simulink model "WPS_system_n_mppt"  (R2019b)
settings: Solver=VariableStepAuto  StartTime=0.0  StopTime=10.0  RelTol=1e-3
undefined symbols (not defined in the file or in its folder): Acid, Lead
libraries: powerlib x17, electricdrivelib x1, powerlib_meascontrol x1, re_lib x1
settings Model: Creator=root  LastModifiedBy=root

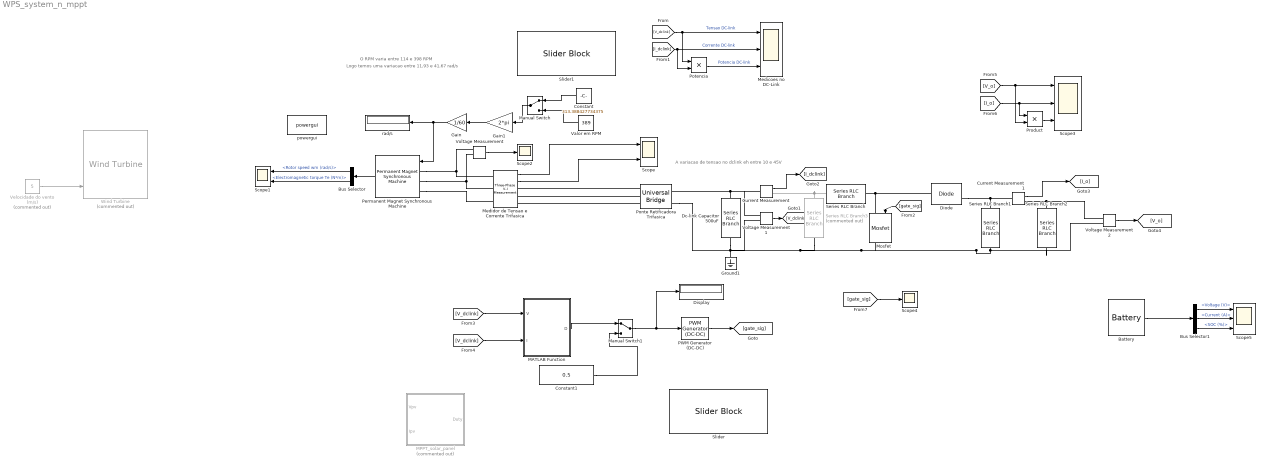
== system WPS_system_n_mppt ==
  note: A variacao de tensao no dclink eh entre 10 e 45V
  note: Logo temos uma variacao entre 11,93 e 41,67 rad/s
  note: O RPM varia entre 114 e 398 RPM
  Battery : electricdrivelib/Extra Sources/Battery  BatType=Lead-Acid  ShowTempParam=off  ThermalPreset=no  ShowAgeParam=off  NomV=12  NomQ=100  SOC=10  Batt_Tr=30  PresetModel=on  MaxQ=104.1667  MinV=9  FullV=13.0658  Dis_rate=20  R=0.0012  Normal_OP=31.0278  expZone="[12.2171     0.333333]"  current=[6.5 13 32.5]  Units=Time  Tci=20  NomT=20  T2=-30  MaxQ2=4.8  FullV2=7.1  Normal_OP2=5.655  expZone2="[6.58           1]"  Rca=0.6  ti=2000  Dp=0  Neq0=0  Tsim=1e6  Ta1=25  Qeol=5.4*0.9  Reol=0.013333*1.2  Char_age=[2.3478, 3]  Dis_age=[2.3478, 10]  N1=1500  N2=10500  N3=1000  N4=1400  Ta2=45  N5=950
      settings: SourceProductName=Simscape Electrical
  Bus Selector : BusSelector  OutputSignals=Rotor speed wm (rad/s),Electromagnetic torque Te (N*m)
  Bus Selector1 : BusSelector  OutputSignals=Voltage (V),Current (A),SOC (%)
  Constant : Constant  Value=313.388427734375
  Constant1 : Constant  Value=0.5
  Current Measurement : powerlib/Measurements/Current Measurement  PhasorSimulation=off  OutputType=Complex  PSBequivalent=0
      settings: SourceProductName=Simscape Electrical
  Current Measurement1 : powerlib/Measurements/Current Measurement  PhasorSimulation=off  OutputType=Complex  PSBequivalent=0
      settings: SourceProductName=Simscape Electrical
  Dc-link Capacitor 500uF : powerlib/Elements/Series RLC Branch  LConnTagsString=__new0  RConnTagsString=__new0  BranchType=C  Resistance=1  Inductance=1e-3  SetiL0=off  InitialCurrent=0  Capacitance=1000e-6  Setx0=off  InitialVoltage=0  Measurements=None
      settings: SourceProductName=Simscape Electrical
  Diode : powerlib/Power Electronics/Diode  Ron=0.001  Lon=0  Vf=0.7  IC=0  UseSnubber=0  Rs=500  Cs=250e-9  Measurements=on
      settings: SourceProductName=Simscape Electrical
  Display : Display
  Gain : Gain  Gain=1/60
  Gain1 : Gain  Gain=2*pi
  Ground1 : powerlib/Elements/Ground  LConnTagsString=a
      settings: SourceProductName=Simscape Electrical
  MATLAB Function : MATLAB Function  TreatAsAtomicUnit=on
  "MPPT_solar_panel " : MATLAB Function  Commented=on  TreatAsAtomicUnit=on
  Manual Switch : ManualSwitch
  Manual Switch1 : ManualSwitch
  Medicoes no DC-Link : Scope  NumInputPorts=3
  Medidor de Tensao e Corrente Trifasica : powerlib/Measurements/Three-Phase V-I Measurement  VoltageMeasurement=phase-to-ground  SetLabelV=off  LabelV=Vabc  Vpu=off  VpuLL=off  CurrentMeasurement=yes  SetLabelI=off  LabelI=Iabc  Ipu=off  Pbase=100e6  Vbase=500e3  OutputType=Complex  PhasorSimulation=off  PSBequivalent=0
      settings: SourceProductName=Simscape Electrical
  Mosfet : powerlib/Power Electronics/Mosfet  Ron=0.1  Lon=0  Rd=0.01  Vfd=0  IC=0  Rs=1e5  Cs=inf  Measurements=on
      settings: SourceProductName=Simscape Electrical
  PWM Generator (DC-DC) : powerlib_meascontrol/Pulse & Signal Generators/PWM Generator (DC-DC)  Fsw=50e3  Ts=0
      settings: SourceProductName=Simscape Electrical
  "Permanent Magnet Synchronous Machine " : powerlib/Machines/Permanent Magnet Synchronous Machine  NbPhases=3  FluxDistribution=Sinusoidal  RotorType=Round  MechanicalLoad=Speed w  PresetModel=No  ShowDetailedParameters=on  MeasurementBus=off  Resistance=0.18  Inductance=8.5e-3  dqInductances=[8.5e-3,8.5e-3]  La=0.000835  MachineConstant=Flux linkage established by magnets (V.s)  Flux=0.186667  VoltageCst=101.5729  TorqueCst=0.84  Flat=120  Mechanical=[0.00038 0.000303448 8]  PolePairs=3  InitialConditions=[0,0, 0,0]  InitialConditions5ph=[0 0 0 0 0 0]  RefAngle=90 degrees behind phase A axis (modified Park)  IterativeDiscreteModel=Trapezoidal non iterative  TsBlock=-1  TsPowergui=0
  Ponte Retificadora Trifasica : powerlib/Power Electronics/Universal Bridge  Arms=3  SnubberResistance=1e4  SnubberCapacitance=100e-6  Device=Diodes  Ron=1e-5  Lon=0  ForwardVoltages="[  0  0  ]"  ForwardVoltage=0  GTOparameters=[ 10e-6 , 20e-6 ]  IGBTparameters=[ 1e-6 , 2e-6 ]  Measurements=None  Measurements_2=None  converterType=Rectifier
      settings: SourceProductName=Simscape Electrical
  Potencia : Product
  Product : Product
  Scope : Scope  NumInputPorts=2
  Scope1 : Scope  NumInputPorts=2
  Scope2 : Scope
  Scope3 : Scope  NumInputPorts=3
  Scope4 : Scope
  Scope5 : Scope  NumInputPorts=3
  Series RLC Branch : powerlib/Elements/Series RLC Branch  LConnTagsString=__new0  RConnTagsString=__new0  BranchType=L  Resistance=1  Inductance=2.7e-3  SetiL0=off  InitialCurrent=0  Capacitance=1e-6  Setx0=off  InitialVoltage=0  Measurements=None
      settings: SourceProductName=Simscape Electrical
  Series RLC Branch1 : powerlib/Elements/Series RLC Branch  LConnTagsString=__new0  RConnTagsString=__new0  BranchType=RC  Resistance=1e-4  Inductance=1e-3  SetiL0=off  InitialCurrent=0  Capacitance=1000e-6  Setx0=off  InitialVoltage=0  Measurements=None
      settings: SourceProductName=Simscape Electrical
  Series RLC Branch2 : powerlib/Elements/Series RLC Branch  LConnTagsString=__new0  RConnTagsString=__new0  BranchType=R  Resistance=10  Inductance=1e-3  SetiL0=off  InitialCurrent=0  Capacitance=1000e-6  Setx0=off  InitialVoltage=0  Measurements=None
      settings: SourceProductName=Simscape Electrical
  Series RLC Branch3 : powerlib/Elements/Series RLC Branch  Commented=on  LConnTagsString=__new0  RConnTagsString=__new0  BranchType=R  Resistance=10  Inductance=1e-3  SetiL0=off  InitialCurrent=0  Capacitance=1000e-6  Setx0=off  InitialVoltage=0  Measurements=None
      settings: SourceProductName=Simscape Electrical
  Slider : SliderBlock  ScaleMax=1
  Slider1 : SliderBlock  ScaleMin=114  ScaleMax=389
  Valor em RPM : Constant  Value=389
  Velocidade do vento (m/s) : Constant  Commented=on  Value=5
  Voltage Measurement : powerlib/Measurements/Voltage Measurement  PhasorSimulation=off  OutputType=Complex  PSBequivalent=0
      settings: SourceProductName=Simscape Electrical
  Voltage Measurement1 : powerlib/Measurements/Voltage Measurement  PhasorSimulation=off  OutputType=Complex  PSBequivalent=0
      settings: SourceProductName=Simscape Electrical
  Voltage Measurement2 : powerlib/Measurements/Voltage Measurement  PhasorSimulation=off  OutputType=Complex  PSBequivalent=0
      settings: SourceProductName=Simscape Electrical
  Wind Turbine : re_lib/Wind Generation/Wind Turbine  Commented=on  Pnom=1.1e3  Pelec_base=1.1e3/0.9  wind_base=5  P_wind_base=0.8  speed_nom=1  pitch_angle=0  c1_c6="[0.51763          116          0.4            5           21     0.006795]"  cp_nom=0.48  lambda_nom=8.1
      settings: SourceProductName=Simscape Electrical  SourceProductBaseCode=PS
  powergui : powerlib/powergui  Priority=1  SimulationMode=Discrete  SampleTime=10e-6  frequency=60  Iterations=50  frequencyindice=0  Pbase=100e6  ErrMax=1e-4  UnitsV=kV  UnitsW=MW  buscounter=0  FunctionMessages=off  echomessages=off  EnableUseOfTLC=off  CurrentSourceSwitches=off  DisableSnubberDevices=off  DisableRonSwitches=off  DisableVfSwitches=off  DisplayEquations=off  AutomaticDiscreteSolvers=off  SolverType=Tustin/Backward Euler (TBE)  Interpol=off  ExternalGateDelay=off  methode=off  Ts=100  x0status=blocks  SPID=on  SwTol=0  HookPort=off  NonlinearTolerance=1e-4  nMaxIteration=100  ContinueOnMaxIteration=off  RestoreLinks=warning  ResistiveCurrentMeasurement=off  Frange=[0:2:500]  Ylog=off  Xlog=on  ShowGrid=off  save=off  variable=ZData  structure=0  ZoomFFT=off  StartTime=0.0  cycles=1  DisplayStyle=1  fundamental=60  FreqAxis=off  MaxFrequency=1000  frequencyindicesteady=1  RmsSteady=1  display=off
      settings: SourceProductName=Simscape Electrical
  rad/s : Display
  wires:
  Velocidade do vento (m/s)/1 -> Wind Turbine/3
  Medidor de Tensao e Corrente Trifasica/1 -> Scope/1
  Medidor de Tensao e Corrente Trifasica/2 -> Scope/2
  "Permanent Magnet Synchronous Machine "/1 -> Bus Selector/1
  Voltage Measurement/1 -> Scope2/1
  PWM Generator (DC-DC)/1 -> [gate_sig]
  Bus Selector/1 -> Scope1/1  "<Rotor speed wm (rad/s)>"
  Bus Selector/2 -> Scope1/2  "<Electromagnetic torque Te (N*m)>"
  Gain1/1 -> Gain/1
  Gain/1 -> rad/s/1, "Permanent Magnet Synchronous Machine "/1
  Valor em RPM/1 -> Manual Switch/2
  Manual Switch/1 -> Gain1/1
  Voltage Measurement1/1 -> [V_dclink]
  Current Measurement/1 -> [I_dclink]
  [V_dclink] -> Medicoes no DC-Link/1, Potencia/1  "Tensao DC-link"
  [I_dclink] -> Medicoes no DC-Link/2, Potencia/2  "Corrente DC-link"
  Potencia/1 -> Medicoes no DC-Link/3  "Potencia DC-link"
  [gate_sig] -> Mosfet/1
  Current Measurement1/1 -> [I_o]
  Voltage Measurement2/1 -> [V_o]
  [V_o] -> Product/2, Scope3/1
  [I_o] -> Product/1, Scope3/2
  Product/1 -> Scope3/3
  [gate_sig] -> Scope4/1
  [V_dclink] -> MATLAB Function/1(V)
  [V_dclink] -> MATLAB Function/2(I)
  Manual Switch1/1 -> Display/1, PWM Generator (DC-DC)/1
  MATLAB Function/1(D) -> Manual Switch1/1
  Constant1/1 -> Manual Switch1/2
  Constant/1 -> Manual Switch/1
  Battery/1 -> Bus Selector1/1
  Bus Selector1/2 -> Scope5/2  "<Current (A)>"
  Bus Selector1/1 -> Scope5/1  "<Voltage (V)>"
  Bus Selector1/3 -> Scope5/3  "<SOC (%)>"
  connections:
  "Permanent Magnet Synchronous Machine "/LConn1 -- Voltage Measurement/LConn1 -- Medidor de Tensao e Corrente Trifasica/LConn1
  "Permanent Magnet Synchronous Machine "/LConn2 -- Medidor de Tensao e Corrente Trifasica/LConn2 -- Voltage Measurement/LConn2
  "Permanent Magnet Synchronous Machine "/LConn3 -- Medidor de Tensao e Corrente Trifasica/LConn3
  Ponte Retificadora Trifasica/LConn1 -- Medidor de Tensao e Corrente Trifasica/RConn1
  Ponte Retificadora Trifasica/LConn2 -- Medidor de Tensao e Corrente Trifasica/RConn2
  Ponte Retificadora Trifasica/LConn3 -- Medidor de Tensao e Corrente Trifasica/RConn3
  Ground1/LConn1 -- Ponte Retificadora Trifasica/RConn2 -- Voltage Measurement1/LConn2 -- Voltage Measurement2/LConn2 -- Series RLC Branch2/RConn1 -- Series RLC Branch1/RConn1 -- Mosfet/RConn1 -- Series RLC Branch3/RConn1 -- Dc-link Capacitor 500uF/RConn1
  Dc-link Capacitor 500uF/LConn1 -- Current Measurement/LConn1 -- Voltage Measurement1/LConn1 -- Ponte Retificadora Trifasica/RConn1
  Mosfet/LConn1 -- Diode/LConn1 -- Series RLC Branch/RConn1
  Diode/RConn1 -- Current Measurement1/LConn1 -- Series RLC Branch1/LConn1
  Current Measurement1/RConn1 -- Series RLC Branch2/LConn1 -- Voltage Measurement2/LConn1
  Series RLC Branch3/LConn1 -- Series RLC Branch/LConn1 -- Current Measurement/RConn1

== matlab function WPS_system_n_mppt/MPPT_solar_panel  ==
  data: Vpv input; Duty output; Ipv input
% Codigo para algoritmo MPPT pertubation and observation
% para o painel fotovoltaico.

function Duty = MPPT_solar_panel(Vpv, Ipv)


    %% Declaramos as variaveis do tipo persistent de forma que os valores 
    % fiquem armazenados mesmo com o término da função
    
    persistent Vpv_old Ppv_old Duty_old
    
    % Inicializacao das variaveis
    if isempty(Duty_old)
       Duty_old = 0.5;
       Ppv_old = 0;
       Vpv_old = 0;
    end
    
    Duty_var = 125e-6;           % Delta de variacao a cada iteracao
    
    
    % Calculo do valor de potencia
    
    Ppv = Vpv * Ipv;
    
    %% Inicializacao da comparacao
    
    if ((Ppv - Ppv_old) ~= 0)
       if ((Ppv - Ppv_old) < 0) 
            if ((Vpv - Vpv_old) < 0)
                Duty = Duty_old - Duty_var;
            else 
                Duty = Duty_old + Duty_var;
            end
       else 
           if ((Vpv - Vpv_old) < 0)
                Duty = Duty_old + Duty_var;
           else 
               Duty = Duty_old - Duty_var;
           end
       end
    else 
        
        Duty = Duty_old;
        
    end
    
    if (Duty > 1)
        Duty = 1.0;
    elseif Duty < 0
        Duty = 0.0;
    end 
    
    Ppv_old = Ppv;
    Vpv_old = Vpv;
    Duty_old = Duty;    
end

== matlab function WPS_system_n_mppt/MATLAB Function ==
  data: V input; D output; I input
% PO algoritm for wind power system

% This function receive voltage and current from dc link
% Dc link is the point following the filter capacitor for rectifier


function D = MPPT_WDS(V, I)


% primeiro declaramos as variaveis

persistent V_old P_old;

if isempty(P_old)
    V_old= 50;
    P_old=100;
end

P = V*I;

dP = P-P_old;
dv = V-V_old;

delta = 0.01;

if (dP~=0)
    if (dP>0)
        if (dv>0)
            V_mppt = V_old + delta;
        else 
            V_mppt = V_old - delta;
        end
    else
        if (dv>0)
            V_mppt = V_old - delta;
        else
            V_mppt = V_old + delta;
        end
    end
else 
    V_mppt = V_old;
end

D = 1- V_mppt/100;

P_old = P;
V_old = V_mppt;
end
